simulink model "task1_simulink"  (Simulink 7.3)
settings: Solver=ode45  StartTime=0.0  StopTime=10.0  RelTol=1e-3
settings Model: Creator=Natalia  LastModifiedBy=Natalia

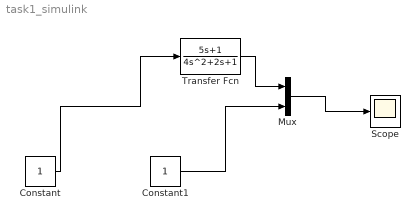
== system task1_simulink ==
  Constant : Constant  OutDataType=fixdt(1, 16)  OutScaling=2^0
  Constant1 : Constant  OutDataType=fixdt(1, 16)  OutScaling=2^0
  Mux : Mux  Inputs=2
  Scope : Scope
  Transfer Fcn : TransferFcn  Numerator=[5,1]  Denominator=[4,2,1]
  wires:
  Constant/1 -> Transfer Fcn/1
  Transfer Fcn/1 -> Mux/1
  Mux/1 -> Scope/1
  Constant1/1 -> Mux/2
